simulink model "ResearchPaper2Fig11"  (R2015b)
settings: Solver=VariableStepAuto  StartTime=0.0  StopTime=10.0  RelTol=1e-3
libraries: xbsIndex_r4 x44, dspvision x1, dspsrcs4 x1
settings Model: Creator=barna  LastModifiedBy=barna

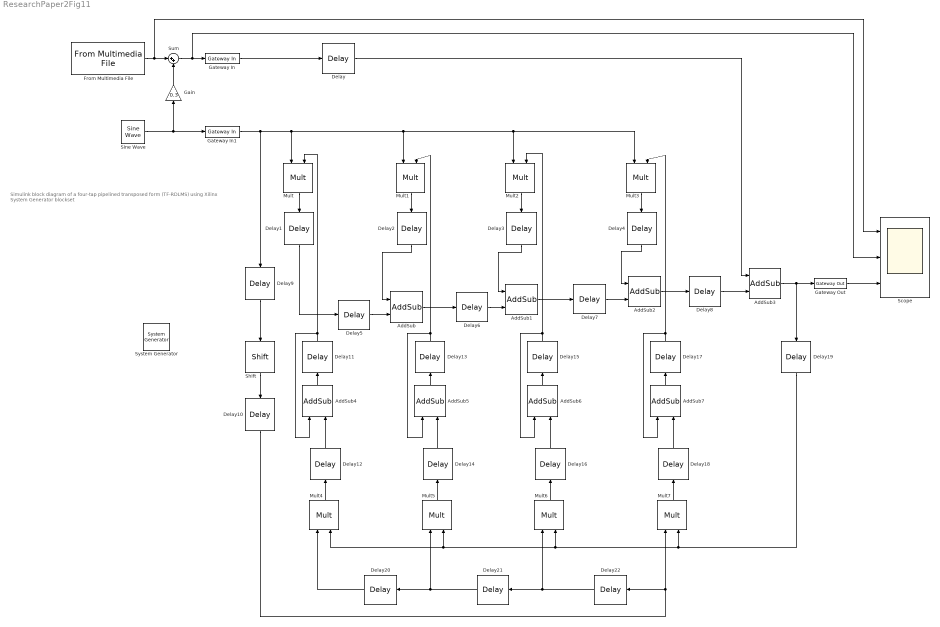
== system ResearchPaper2Fig11 ==
  note: Simulink block diagram of a four-tap pipelined transposed form (TF-RDLMS) using Xilinx System Generator blockset
  " System Generator" : xbsIndex_r4/ System Generator  Tag=genX  xilinxfamily=kintex7  part=xc7k325t  speed=-3  package=fbg676  synthesis_tool=Vivado  clock_wrapper=Clock Enables  directory=./netlist  proj_type=Vivado  Synth_file=Vivado Synthesis Defaults  Impl_file=Vivado Implementation Defaults  testbench=off  simulink_period=1  sysclk_period=10  dcm_input_clock_period=10  incr_netlist=off  trim_vbits=Everywhere in SubSystem  dbl_ovrd=According to Block Masks  core_generation=According to Block Masks  run_coregen=off  deprecated_control=off  eval_field=0  block_type=sysgen
  AddSub{,1..2,4..7} (7 alike) : xbsIndex_r4/AddSub  mode=Addition  use_carryin=off  use_carryout=off  en=off  latency=0  precision=Full  arith_type=Unsigned  n_bits=16  bin_pt=14  quantization=Truncate  overflow=Wrap  use_behavioral_HDL=off  hw_selection=Fabric  pipelined=off  dbl_ovrd=off  block_type=addsub
  AddSub3 : xbsIndex_r4/AddSub  mode=Subtraction  use_carryin=off  use_carryout=off  en=off  latency=0  precision=Full  arith_type=Unsigned  n_bits=16  bin_pt=14  quantization=Truncate  overflow=Wrap  use_behavioral_HDL=off  hw_selection=Fabric  pipelined=off  dbl_ovrd=off  block_type=addsub
  Delay : xbsIndex_r4/Delay  rst=off  infoeditControl=Selection of Reset will increase slice count due to use of real FFs and instead of SRLs  en=off  latency=2  reg_retiming=off  dbl_ovrd=off  block_type=delay
  Delay{1..8,10..22} (21 alike) : xbsIndex_r4/Delay  rst=off  infoeditControl=Selection of Reset will increase slice count due to use of real FFs and instead of SRLs  en=off  latency=1  reg_retiming=off  dbl_ovrd=off  block_type=delay
  Delay9 : xbsIndex_r4/Delay  rst=off  infoeditControl=Selection of Reset will increase slice count due to use of real FFs and instead of SRLs  en=off  latency=2  reg_retiming=off  dbl_ovrd=off  block_type=delay
  From Multimedia File : dspvision/From Multimedia File  inputFilename=vipmen.avi  loop=on  numPlays=inf  outputStreams=Video only  videoDataType=single  audioDataType=int16  inheritSampleTime=on  userDefinedSampleTime=1/30  noAudioOutput=off  isIntensityVideo=off  fourcc=RGB  colorVideoFormat=One multidimensional signal  outputEOF=off  dataOrg=Column-major  audioFrameSize=1024  computeAudioFrameSize=off  outSamplingMode=Sample based
  Gain : Gain  Gain=0.3
  Gateway In : xbsIndex_r4/Gateway In  gui_display_data_type=Fixed-point  arith_type="Signed  (2's comp)"  n_bits=16  bin_pt=14  preci_type=Single  exp_width=8  frac_width=24  rows=1  columns=1  quantization="Round  (unbiased: +/- Inf)"  overflow=Saturate  period=1  UseAsADC=off  ADCChannel='1'  interface=None  automatic_assignment=on  address_offset=hex2dec('00')  intf_name=''  intf_description=''  default_value=0  timing_constraint=None  locs_specified=off  LOCs={}  io_standard={}  inherit_from_input=off  hdl_port=on  dbl_ovrd=off  block_type=gatewayin
  Gateway In1 : xbsIndex_r4/Gateway In  gui_display_data_type=Fixed-point  arith_type="Signed  (2's comp)"  n_bits=16  bin_pt=14  preci_type=Single  exp_width=8  frac_width=24  rows=1  columns=1  quantization="Round  (unbiased: +/- Inf)"  overflow=Saturate  period=1  UseAsADC=off  ADCChannel='1'  interface=None  automatic_assignment=on  address_offset=hex2dec('00')  intf_name=''  intf_description=''  default_value=0  timing_constraint=None  locs_specified=off  LOCs={}  io_standard={}  inherit_from_input=off  hdl_port=on  dbl_ovrd=off  block_type=gatewayin
  Gateway Out : xbsIndex_r4/Gateway Out  inherit_from_input=off  hdl_port=on  rows=1  columns=1  UseAsDAC=off  DACChannel='1'  interface=None  automatic_assignment=on  address_offset=hex2dec('00')  intf_name=''  intf_description=''  timing_constraint=None  locs_specified=off  LOCs={}  io_standard={}  block_type=gatewayout
  Mult{,1..7} (8 alike) : xbsIndex_r4/Mult  precision=Full  arith_type="Signed  (2's comp)"  n_bits=16  bin_pt=14  quantization=Truncate  overflow=Wrap  en=off  latency=0  use_behavioral_HDL=off  opt=Speed  use_embedded=on  optimum_pipeline=off  pipeline=on  dbl_ovrd=off  use_rpm=on  placement_style=Triangular  block_type=mult
  Scope : Scope  NumInputPorts=3
  Shift : xbsIndex_r4/Shift  shift_dir=Right  shift_bits=4  en=off  latency=0  precision=Full  arith_type="Signed  (2's comp)"  n_bits=16  bin_pt=14  quantization=Truncate  overflow=Wrap  dbl_ovrd=off  block_type=shift
  Sine Wave : dspsrcs4/Sine Wave  Amplitude=1  Frequency=100  Phase=0  SampleMode=Discrete  OutComplex=Real  CompMethod=Trigonometric fcn  TableSize=Speed  SampleTime=1/1000  SamplesPerFrame=1  ResetState=Restart at time zero  OutputFrames=off  dataType=double  wordLen=16  udDataType=sfix(16)  fracBitsMode=Best precision  numFracBits=15  OutDataTypeStr=double  LastOutDataTypeStr=double
  Sum : Sum  Inputs=|++
  wires:
  Sine Wave/1 -> Gain/1, Gateway In1/1
  Gain/1 -> Sum/2
  Sum/1 -> Gateway In/1, Scope/2
  Gateway In/1 -> Delay/1
  Gateway In1/1 -> Mult/1, Mult1/1, Mult3/1, Mult2/1, Delay9/1
  Mult/1 -> Delay1/1
  Mult1/1 -> Delay2/1
  Mult2/1 -> Delay3/1
  Mult3/1 -> Delay4/1
  Delay1/1 -> Delay5/1
  Delay2/1 -> AddSub/1
  Delay5/1 -> AddSub/2
  AddSub/1 -> Delay6/1
  Delay6/1 -> AddSub1/2
  Delay3/1 -> AddSub1/1
  AddSub1/1 -> Delay7/1
  Delay7/1 -> AddSub2/2
  Delay4/1 -> AddSub2/1
  AddSub2/1 -> Delay8/1
  Delay8/1 -> AddSub3/2
  Delay/1 -> AddSub3/1
  AddSub3/1 -> Delay19/1, Gateway Out/1
  Delay9/1 -> Shift/1
  Shift/1 -> Delay10/1
  Delay11/1 -> AddSub4/1, Mult/2
  AddSub4/1 -> Delay11/1
  Delay12/1 -> AddSub4/2
  AddSub5/1 -> Delay13/1
  Delay14/1 -> AddSub5/2
  Delay13/1 -> AddSub5/1, Mult1/2
  AddSub6/1 -> Delay15/1
  Delay16/1 -> AddSub6/2
  Delay15/1 -> AddSub6/1, Mult2/2
  AddSub7/1 -> Delay17/1
  Delay18/1 -> AddSub7/2
  Delay17/1 -> AddSub7/1, Mult3/2
  Mult4/1 -> Delay12/1
  Mult5/1 -> Delay14/1
  Mult6/1 -> Delay16/1
  Mult7/1 -> Delay18/1
  Delay19/1 -> Mult7/2, Mult6/2, Mult5/2, Mult4/2
  Delay20/1 -> Mult4/1
  Delay21/1 -> Delay20/1, Mult5/1
  Delay22/1 -> Mult6/1, Delay21/1
  Delay10/1 -> Mult7/1, Delay22/1
  From Multimedia File/1 -> Scope/1, Sum/1
  Gateway Out/1 -> Scope/3
